simulink model "group2_assignment2_pacemaker_demofile"  (R2023b)
settings: Solver=FixedStepAuto  StartTime=0.0  StopTime=10  FixedStep=1e-3  RelTol=1e-3  EnableMultiTasking=on
model workspace (MAT data in the model file):
  IC = 60
  j = 80
undefined symbols (not defined in the file): D0, D1, D10, D11, D12, D13, D2, D3, D4, D5, D6, D7, D8, D9, PTA0, PTA1, PTA2, PTB23, PTB9, PTC16, PTC17, PTC2, PTC3, PTC4, PTD0, PTD1, PTD2, PTD3
libraries: frdmk64flib x15, dspstat3 x3
settings Model: SimulationMode=external  ExtModeTrigDuration=5  Creator=stivb  LastModifiedBy=bardiased
settings OptimizationCC: EnhancedBackFolding=on  PassReuseOutputArgsAs=Individual arguments  ZeroExternalMemoryAtStartup=off  ZeroInternalMemoryAtStartup=off  MaxStackSize=64  OptimizeBlockOrder=speed  DifferentSizesBufferReuse=on  OptimizationCustomize=off  EfficientTunableParamExpr=on
settings DebuggingCC: ParameterTunabilityLossMsg=error
settings HardwareCC: ProdBitPerPointer=32  ProdBitPerSizeT=32  ProdBitPerPtrDiffT=32  ProdLargestAtomicInteger=Long  ProdLargestAtomicFloat=Double  ProdWordSize=32  ProdHWDeviceType=ARM Compatible->ARM Cortex
settings RTWCC: Description=Embedded Coder  SystemTargetFile=ert.tlc  HardwareBoard=NXP FRDM-K64F  TLCOptions="-aInlineSetEventsForThisBaseRateFcn=TLC_FALSE -aSuppressMultiTaskScheduler=TLC_FALSE  -aRateBasedStepFcn=0"  TemplateMakefile=ert_default_tmf  Toolchain=GNU Tools for ARM Embedded Processors
settings CodeAppCC: ForceParamTrailComments=on  IgnoreCustomStorageClasses=off  OperatorAnnotations=on  SimulinkDataObjDesc=on  SFDataObjDesc=on  InsertBlockDesc=on
settings ERTTargetCC: SupportContinuousTime=on  SupportVariableSizeSignals=on  ExtModeTransport=4  ExtModeMexFile=sendToCommService

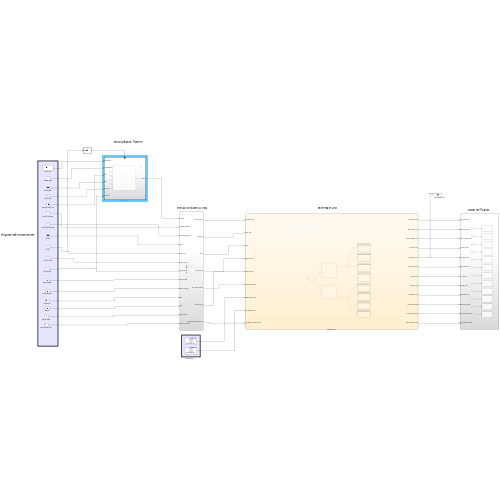
[thumbnail: Simulink's stored preview of the top-level diagram]
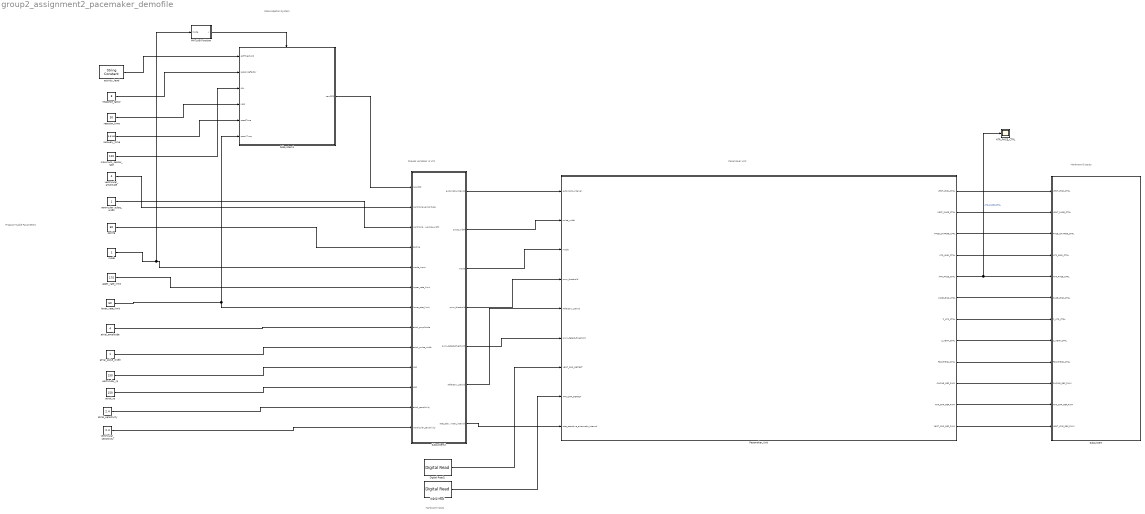
== system group2_assignment2_pacemaker_demofile ==
  note: Rate Adaption System
  note: Hardware inputs
  note: Pseudo variables (4 VM)
  note: Programmable Parameters
  note: Pacemaker Unit
  note: Hardware Outputs
  ATR_PACE_CTRL : Scope
  Digital Read : frdmk64flib/Digital Read  Whichpin=PTC16 (D0)  SampleTime=-1
  Digital Read1 : frdmk64flib/Digital Read  Whichpin=PTC17 (D1)  SampleTime=-1
  MATLAB Function : MATLAB Function  TreatAsAtomicUnit=on
  Pacemaker_Unit : Stateflow chart  TreatAsAtomicUnit=on
      settings: PortSchema="{\"entries\":[{\"content\":{\"sides\":[{\"content\":{\"connectorIds\":[\"In1\",\"In2\",\"In3\",\"In4\",\"In5\",\"In6\",\"In8\",\"In7\",\"In9\"]},\"type\":\"ConnectorPlacement.EquallySpacedRectSide\",\"uuid\":\"c8cba9b3-707c-4f69-ad8c-9d5fbaa12caa\"},{\"content\":{\"connectorIds\":[\"Out1\",\"Out2\",\"Out3\",\"Out4\",\"Out5\",\"Out6\",\"Out7\",\"Out8\",\"Out9\",\"Out10\",\"Out11\",\"Out12\"],\"side\":\"RIGHT\"},\"type\":\"ConnectorPlacement.EquallySpacedRectSide\",\"uuid\":\"918aa1e0-aae1-41d7-a74d-0a72155b1f75\"},{\"content\":{\"side\":\"TOP\"},\"type\":\"ConnectorPlacement.EquallySpacedRectSide\",\"uuid\":\"877803b3-29d8-4e86-807a-7bf9f59cc519\"}]},\"type\":\"ConnectorPlacement.EquallySpacedConnector\",\"uuid\":\"1e148aae-cf3c-4ae1-bc6b-9e679c8c5f2a\"}],\"packageUris\":[\"http://schema.mathworks.com/mf0/Connector/R2020b\"],\"version\":\"1.0\"}"
  Subsystem : Subsystem
  Subsystem1 : Subsystem
  Subsystem2 : Subsystem
  activity_level : StringConstant  String="\"V-Low\""
  atrial_amplitude : Constant  Value=4
  atrial_pulse_width : Constant
  atrial_rp : Constant  Value=150
  atrial_sensitivity : Constant  Value=2.4
  lower_rate_limit : Constant  Value=60
  maximum_sensor_rate : Constant  Value=120
  mode : Constant
  pacing : Constant  Value=60
  reaction_time : Constant  Value=30
  recovery_time : Constant  Value=0.5*60
  response_factor : Constant  Value=8
  upper_rate_limit : Constant  Value=175
  ventricular_amplitude : Constant  Value=4
  ventricular_pulse_width : Constant
  ventricular_rp : Constant  Value=150
  ventricular_sensitivity : Constant  Value=2.4
  wires:
  mode/1 -> MATLAB Function/1(mode), Subsystem2/5(mode_input)
  ventricular_amplitude/1 -> Subsystem2/2(ventricular_amplitude)
  atrial_amplitude/1 -> Subsystem2/8(atrial_amplitude)
  atrial_pulse_width/1 -> Subsystem2/9(atrial_pulse_width)
  lower_rate_limit/1 -> Subsystem1/6(recovTime), Subsystem2/7(lower_rate_limit)
  upper_rate_limit/1 -> Subsystem2/6(upper_rate_limit)
  ventricular_pulse_width/1 -> Subsystem2/3(ventricular_pulse_width)
  pacing/1 -> Subsystem2/4(pacing)
  Subsystem2/1(automatic_interval) -> Pacemaker_Unit/1(automatic_interval)
  Subsystem2/2(pulse_width) -> Pacemaker_Unit/2(pulse_width)
  Subsystem2/3(mode) -> Pacemaker_Unit/3(mode)
  Subsystem2/4(pwm_threshold) -> Pacemaker_Unit/4(pwm_threshold)
  Subsystem2/6(refractory_period) -> Pacemaker_Unit/5(refractory_period)
  Pacemaker_Unit/1(VENT_GND_CTRL) -> Subsystem/1(VENT_GND_CTRL)
  Pacemaker_Unit/2(VENT_PACE_CTRL) -> Subsystem/2(VENT_PACE_CTRL)
  Pacemaker_Unit/3(PACE_CHARGE_CTRL) -> Subsystem/3(PACE_CHARGE_CTRL)
  Pacemaker_Unit/4(ATR_GND_CTRL) -> Subsystem/4(ATR_GND_CTRL)
  Pacemaker_Unit/5(ATR_PACE_CTRL) -> ATR_PACE_CTRL/1, Subsystem/5(ATR_PACE_CTRL)  "ATR_PACE_CTRL"
  Pacemaker_Unit/6(PACE_GND_CTRL) -> Subsystem/6(PACE_GND_CTRL)
  Pacemaker_Unit/7(Z_ATR_CTRL) -> Subsystem/7(Z_ATR_CTRL)
  Pacemaker_Unit/8(Z_VENT_CTRL) -> Subsystem/8(Z_VENT_CTRL)
  Pacemaker_Unit/9(FRONTEND_CTRL) -> Subsystem/9(FRONTEND_CTRL)
  Pacemaker_Unit/10(PACING_REF_PWM) -> Subsystem/10(PACING_REF_PWM)
  ventricular_rp/1 -> Subsystem2/10(VRP)
  atrial_rp/1 -> Subsystem2/11(ARP)
  Pacemaker_Unit/11(ATR_CMP_REF_PWM) -> Subsystem/11(ATR_CMP_REF_PWM)
  Digital Read/1 -> Pacemaker_Unit/7(ATR_CMP_DETECT)
  Digital Read1/1 -> Pacemaker_Unit/8(VENT_CMP_DETECT)
  atrial_sensitivity/1 -> Subsystem2/12(atrial_sensitivity)
  ventricular_sensitivity/1 -> Subsystem2/13(ventricular_sensitivity)
  Subsystem2/5(pwm_detect_threshold) -> Pacemaker_Unit/6(pwm_detect_threshold)
  Pacemaker_Unit/12(VENT_CMP_REF_PWM) -> Subsystem/12(VENT_CMP_REF_PWM)
  Subsystem2/7(rate_adaptive_automatic_interval) -> Pacemaker_Unit/9(rate_adaptive_automatic_interval)
  activity_level/1 -> Subsystem1/1(actThreshold)
  response_factor/1 -> Subsystem1/2(responseFactor)
  maximum_sensor_rate/1 -> Subsystem1/3(LRL)
  reaction_time/1 -> Subsystem1/4(MSR)
  recovery_time/1 -> Subsystem1/5(reactTime)
  Subsystem1/1(newCPR) -> Subsystem2/1(newCPR)
  MATLAB Function/1(y) -> Subsystem1/Enable

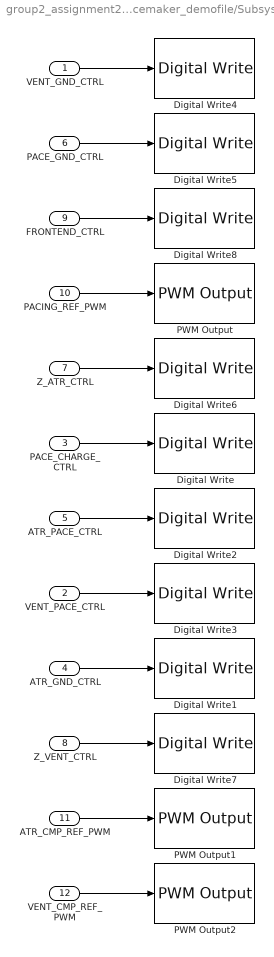
== system group2_assignment2_pacemaker_demofile/Subsystem ==
  VENT_GND_CTRL : Inport
  VENT_PACE_CTRL : Inport  Port=2
  PACE_CHARGE_CTRL : Inport  Port=3
  ATR_GND_CTRL : Inport  Port=4
  ATR_PACE_CTRL : Inport  Port=5
  PACE_GND_CTRL : Inport  Port=6
  Z_ATR_CTRL : Inport  Port=7
  Z_VENT_CTRL : Inport  Port=8
  FRONTEND_CTRL : Inport  Port=9
  PACING_REF_PWM : Inport  Port=10
  ATR_CMP_REF_PWM : Inport  Port=11
  VENT_CMP_REF_PWM : Inport  Port=12
  Digital Write : frdmk64flib/Digital Write  Whichpin=PTB9 (D2)
  Digital Write1 : frdmk64flib/Digital Write  Whichpin=PTD2 (D11)
  Digital Write2 : frdmk64flib/Digital Write  Whichpin=PTA0 (D8)
  Digital Write3 : frdmk64flib/Digital Write  Whichpin=PTC4 (D9)
  Digital Write4 : frdmk64flib/Digital Write  Whichpin=PTD3 (D12)
  Digital Write5 : frdmk64flib/Digital Write  Whichpin=PTD0 (D10)
  Digital Write6 : frdmk64flib/Digital Write  Whichpin=PTB23 (D4)
  Digital Write7 : frdmk64flib/Digital Write  Whichpin=PTC3 (D7)
  Digital Write8 : frdmk64flib/Digital Write  Whichpin=PTD1 (D13)
  PWM Output : frdmk64flib/PWM Output  Whichpin=PTA2 (D5)  InitialFrequency=2000  InitialDutyCycle=0
  PWM Output1 : frdmk64flib/PWM Output  Whichpin=PTC2 (D6)  InitialFrequency=2000  InitialDutyCycle=0
  PWM Output2 : frdmk64flib/PWM Output  Whichpin=PTA1 (D3)  InitialFrequency=2000  InitialDutyCycle=0
  wires:
  Z_ATR_CTRL/1 -> Digital Write6/1
  VENT_PACE_CTRL/1 -> Digital Write3/1
  FRONTEND_CTRL/1 -> Digital Write8/1
  PACING_REF_PWM/1 -> PWM Output/1
  ATR_PACE_CTRL/1 -> Digital Write2/1
  Z_VENT_CTRL/1 -> Digital Write7/1
  VENT_GND_CTRL/1 -> Digital Write4/1
  PACE_CHARGE_CTRL/1 -> Digital Write/1
  ATR_GND_CTRL/1 -> Digital Write1/1
  PACE_GND_CTRL/1 -> Digital Write5/1
  ATR_CMP_REF_PWM/1 -> PWM Output1/1
  VENT_CMP_REF_PWM/1 -> PWM Output2/1

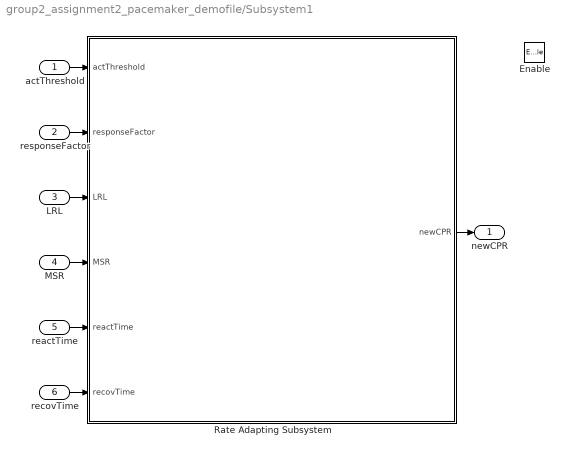
== system group2_assignment2_pacemaker_demofile/Subsystem1 ==
  actThreshold : Inport
  responseFactor : Inport  Port=2
  LRL : Inport  Port=3
  MSR : Inport  Port=4
  reactTime : Inport  Port=5
  recovTime : Inport  Port=6
  Enable : EnablePort
  Rate Adapting Subsystem : Subsystem
  newCPR : Outport
  wires:
  MSR/1 -> Rate Adapting Subsystem/4(MSR)
  reactTime/1 -> Rate Adapting Subsystem/5(reactTime)
  LRL/1 -> Rate Adapting Subsystem/3(LRL)
  Rate Adapting Subsystem/1(newCPR) -> newCPR/1
  responseFactor/1 -> Rate Adapting Subsystem/2(responseFactor)
  recovTime/1 -> Rate Adapting Subsystem/6(recovTime)
  actThreshold/1 -> Rate Adapting Subsystem/1(actThreshold)

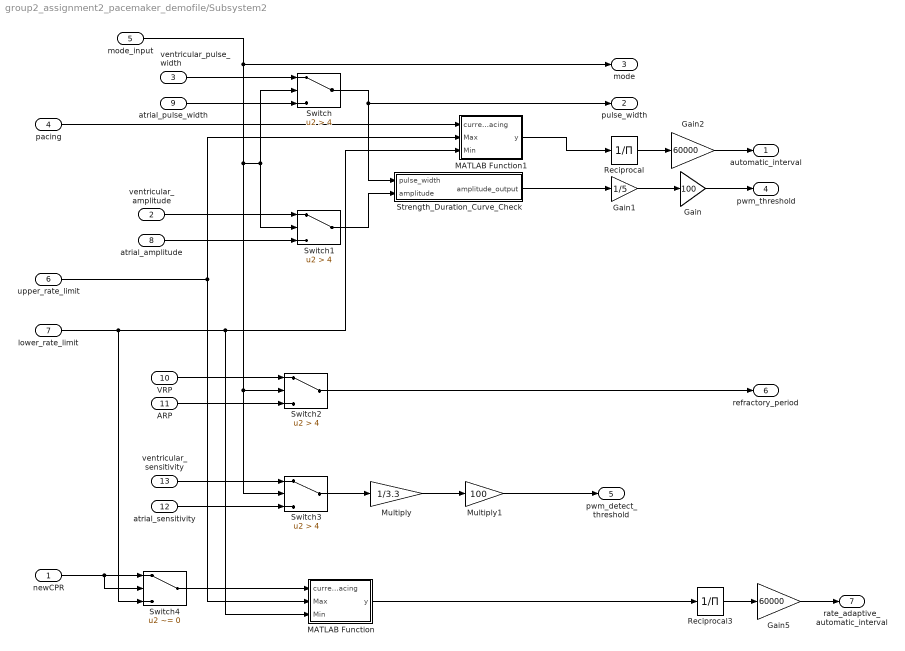
== system group2_assignment2_pacemaker_demofile/Subsystem2 ==
  newCPR : Inport
  ventricular_amplitude : Inport  Port=2
  ventricular_pulse_width : Inport  Port=3
  pacing : Inport  Port=4
  mode_input : Inport  Port=5
  upper_rate_limit : Inport  Port=6
  lower_rate_limit : Inport  Port=7
  atrial_amplitude : Inport  Port=8
  atrial_pulse_width : Inport  Port=9
  VRP : Inport  Port=10
  ARP : Inport  Port=11
  atrial_sensitivity : Inport  Port=12
  ventricular_sensitivity : Inport  Port=13
  Gain : Gain  Gain=100
  Gain1 : Gain  Gain=1/5
  Gain2 : Gain  Gain=60000
  Gain5 : Gain  Gain=60000
  MATLAB Function : MATLAB Function  TreatAsAtomicUnit=on
  MATLAB Function1 : MATLAB Function  TreatAsAtomicUnit=on
  Multiply : Gain  Gain=1/3.3
  Multiply1 : Gain  Gain=100
  Reciprocal : Product  Inputs=/
  Reciprocal3 : Product  Inputs=/
  Strength_Duration_Curve_Check : Stateflow chart  TreatAsAtomicUnit=on
  Switch{,1..3} (4 alike) : Switch  Criteria=u2 > Threshold  Threshold=4  SaturateOnIntegerOverflow=off  InputSameDT=off
  Switch4 : Switch  Criteria=u2 ~= 0  Threshold=4  SaturateOnIntegerOverflow=off  InputSameDT=off
  automatic_interval : Outport
  pulse_width : Outport  Port=2
  mode : Outport  Port=3
  pwm_threshold : Outport  Port=4
  pwm_detect_threshold : Outport  Port=5
  refractory_period : Outport  Port=6
  rate_adaptive_automatic_interval : Outport  Port=7
  wires:
  Gain1/1 -> Gain/1
  upper_rate_limit/1 -> MATLAB Function1/2(Max), MATLAB Function/2(Max)
  Reciprocal/1 -> Gain2/1
  Gain2/1 -> automatic_interval/1
  Gain/1 -> pwm_threshold/1
  Strength_Duration_Curve_Check/1(amplitude_output) -> Gain1/1
  lower_rate_limit/1 -> Switch4/3, MATLAB Function/3(Min), MATLAB Function1/3(Min)
  Switch1/1 -> Strength_Duration_Curve_Check/2(amplitude)
  Switch/1 -> Strength_Duration_Curve_Check/1(pulse_width), pulse_width/1
  Switch2/1 -> refractory_period/1
  VRP/1 -> Switch2/1
  ARP/1 -> Switch2/3
  ventricular_amplitude/1 -> Switch1/1
  ventricular_pulse_width/1 -> Switch/1
  atrial_pulse_width/1 -> Switch/3
  atrial_amplitude/1 -> Switch1/3
  mode_input/1 -> Switch3/2, Switch2/2, Switch1/2, Switch/2, mode/1
  atrial_sensitivity/1 -> Switch3/3
  ventricular_sensitivity/1 -> Switch3/1
  Switch3/1 -> Multiply/1
  Multiply/1 -> Multiply1/1
  Multiply1/1 -> pwm_detect_threshold/1
  Gain5/1 -> rate_adaptive_automatic_interval/1
  Reciprocal3/1 -> Gain5/1
  newCPR/1 -> Switch4/2, Switch4/1
  Switch4/1 -> MATLAB Function/1(currentPacing)
  MATLAB Function/1(y) -> Reciprocal3/1
  pacing/1 -> MATLAB Function1/1(currentPacing)
  MATLAB Function1/1(y) -> Reciprocal/1

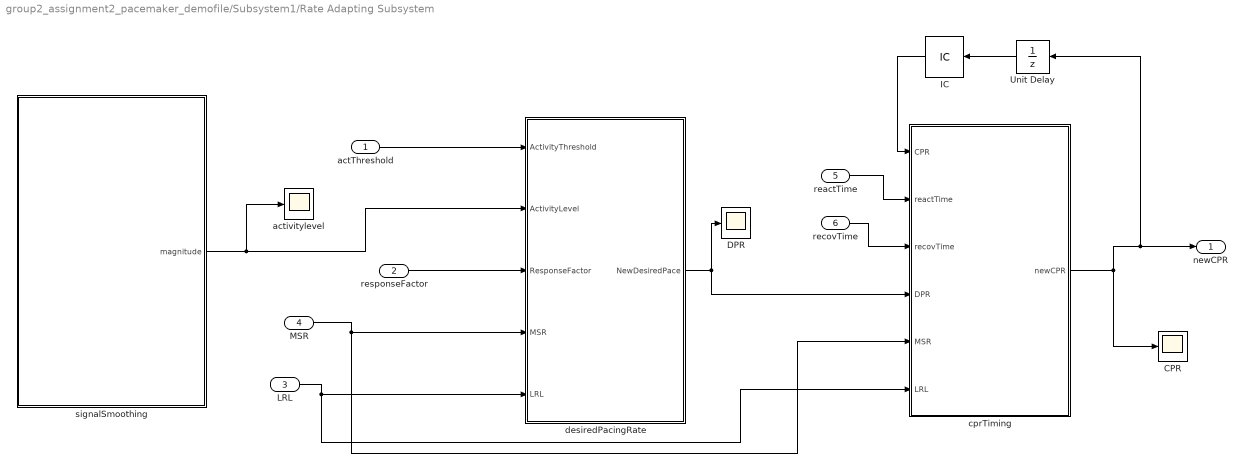
== system group2_assignment2_pacemaker_demofile/Subsystem1/Rate Adapting Subsystem ==
  actThreshold : Inport
  responseFactor : Inport  Port=2
  LRL : Inport  Port=3
  MSR : Inport  Port=4
  reactTime : Inport  Port=5
  recovTime : Inport  Port=6
  CPR : Scope
  DPR : Scope
  IC : InitialCondition  Value=60
  Unit Delay : UnitDelay  SampleTime=-1  HasFrameUpgradeWarning=on
  activitylevel : Scope
  cprTiming : Stateflow chart  TreatAsAtomicUnit=on
  desiredPacingRate : Stateflow chart  TreatAsAtomicUnit=on
  signalSmoothing : Subsystem
  newCPR : Outport
  wires:
  desiredPacingRate/1(NewDesiredPace) -> DPR/1, cprTiming/4(DPR)
  LRL/1 -> desiredPacingRate/5(LRL), cprTiming/6(LRL)
  responseFactor/1 -> desiredPacingRate/3(ResponseFactor)
  MSR/1 -> desiredPacingRate/4(MSR), cprTiming/5(MSR)
  actThreshold/1 -> desiredPacingRate/1(ActivityThreshold)
  cprTiming/1(newCPR) -> Unit Delay/1, newCPR/1, CPR/1
  reactTime/1 -> cprTiming/2(reactTime)
  recovTime/1 -> cprTiming/3(recovTime)
  Unit Delay/1 -> IC/1
  IC/1 -> cprTiming/1(CPR)
  signalSmoothing/1(magnitude) -> activitylevel/1, desiredPacingRate/2(ActivityLevel)

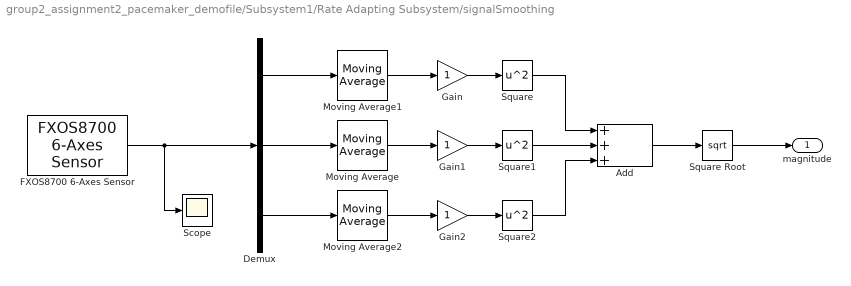
== system group2_assignment2_pacemaker_demofile/Subsystem1/Rate Adapting Subsystem/signalSmoothing ==
  Add : Sum  Inputs=+++
  Demux : Demux  Outputs=3
  FXOS8700 6-Axes Sensor : frdmk64flib/FXOS8700 6-Axes Sensor  Activesensor=Accelerometer only  ODR=800Hz  HybridODR=400Hz  Accelfullrange=-4g to +4g  SampleTime=-1
  Gain : Gain
  Gain1 : Gain
  Gain2 : Gain
  Moving Average : dspstat3/Moving Average  Method=Sliding window  ForgettingFactorPort=off  SpecifyWindowLength=on  WindowLength=4  OverlapLength=3  AllowArbitraryInputLength=off  ForgettingFactor=0.9  SimulateUsing=Code generation
  Moving Average1 : dspstat3/Moving Average  Method=Sliding window  ForgettingFactorPort=off  SpecifyWindowLength=on  WindowLength=4  OverlapLength=3  AllowArbitraryInputLength=off  ForgettingFactor=0.9  SimulateUsing=Code generation
  Moving Average2 : dspstat3/Moving Average  Method=Sliding window  ForgettingFactorPort=off  SpecifyWindowLength=on  WindowLength=4  OverlapLength=3  AllowArbitraryInputLength=off  ForgettingFactor=0.9  SimulateUsing=Code generation
  Scope : Scope
  Square : Math  Operator=square
  Square Root : Sqrt
  Square1 : Math  Operator=square
  Square2 : Math  Operator=square
  magnitude : Outport
  wires:
  Demux/2 -> Moving Average/1
  Moving Average/1 -> Gain1/1
  Demux/1 -> Moving Average1/1
  Moving Average1/1 -> Gain/1
  Demux/3 -> Moving Average2/1
  FXOS8700 6-Axes Sensor/1 -> Scope/1, Demux/1
  Moving Average2/1 -> Gain2/1
  Square Root/1 -> magnitude/1
  Gain/1 -> Square/1
  Gain1/1 -> Square1/1
  Gain2/1 -> Square2/1
  Square/1 -> Add/1
  Square1/1 -> Add/2
  Square2/1 -> Add/3
  Add/1 -> Square Root/1

== stateflow chart group2_assignment2_pacemaker_demofile/Pacemaker_Unit ==
  note: %3CmxGraphModel%3E%3Croot%3E%3CmxCell%20id%3D%220%22%2F%3E%3CmxCell%20id%3D%221%22%20parent%3D%220%22%2F%3E%3CmxCell%20id%3D%222%22%20value%3D%22Assumption%3A%20All%20the%20hazards%20can%20be%20identified%22%20style%3D%22ellipse%3BwhiteSpace%3Dwrap%3Bhtml%3D1%3BfillColor%3D%23CCFFFF%3B%22%20vertex%3D%221%22%20parent%3D%221%22%3E%3CmxGeometry%20x%3D%22370%22%20y%3D%22280%22%20width%3D%22130%22%20height%3D%2280%22%20as%3D%22geometry%22%2F%3E%3C%2FmxCell%3E%3C%2Froot%3E%3C%2FmxGraphModel%3E
  state VOO
    state Charge_C22_Discharge_C21
      entry:
      %Charge C22
      VENT_PACE_CTRL = 0;
      PACE_CHARGE_CTRL = 1;
      %Discharge C21
      VENT_GND_CTRL= 1;
    state ChargeC21_and_DischargeC22
      %Creates the leading edge and sends pulse for X amount of time
      entry:
      PACE_CHARGE_CTRL = 0;
      VENT_GND_CTRL = 0;
      VENT_PACE_CTRL = 1;
      %Recharge pulse is the current in the opposite direction due to C21
    (default) -> VOO.Charge_C22_Discharge_C21
    VOO.Charge_C22_Discharge_C21 -> VOO.ChargeC21_and_DischargeC22 : after(automatic_interval-pulse_width, msec)
    VOO.ChargeC21_and_DischargeC22 -> VOO.Charge_C22_Discharge_C21 : after(pulse_width, msec)
  state VVI
    note: Safe start entry; since hysteresis pacing allows for waiting a period of time longer than the refractory period, we are okay with waiting a refractory period of time before we start pacing. This also ensures that the capacitors are appropriately charged to allow for proper pacing.
    state Refractory_and_charging_ventricle
      entry:
      %Charge C22
      VENT_PACE_CTRL = 0;
      PACE_CHARGE_CTRL = 1;
      %Discharge C21
      VENT_GND_CTRL= 1;
      % Setup sensing pins
      VENT_CMP_REF_PWM = pwm_detect_threshold;
    note: Detected a pace, so go back to refractory state to wait
        | the appropriate refractory time interval
    state Sensing_ventricle
      entry:
      FRONTEND_CTRL = 1;
    state Pacing_ventricle
      entry:
      PACE_CHARGE_CTRL = 0;
      VENT_PACE_CTRL = 1;
      VENT_GND_CTRL = 0;
    (default) -> VVI.Refractory_and_charging_ventricle
    VVI.Refractory_and_charging_ventricle -> VVI.Sensing_ventricle : after(refractory_period, msec)
    VVI.Sensing_ventricle -> VVI.Refractory_and_charging_ventricle [order 1] : [VENT_CMP_DETECT == true]
    VVI.Pacing_ventricle -> VVI.Refractory_and_charging_ventricle : after(pulse_width, msec)
    VVI.Sensing_ventricle -> VVI.Pacing_ventricle [order 2] : after(automatic_interval - refractory_period - pulse_width, msec)
  state Ventricular_Safe_State
    entry: %Safe State
    ATR_PACE_CTRL = 0;
    VENT_PACE_CTRL=0;
    PACING_REF_PWM = pwm_threshold;
    PACE_CHARGE_CTRL=0;
    PACE_GND_CTRL = 1;
    VENT_PACE_CTRL=0;
    Z_ATR_CTRL=0;
    Z_VENT_CTRL=0;
    ATR_PACE_CTRL=0;
    ATR_GND_CTRL=0;
    VENT_GND_CTRL=1;
    FRONTEND_CTRL=0;
  state VOOR
    state Charge_C22_Discharge_C21
      entry:
      %Charge C22
      VENT_PACE_CTRL = 0;
      PACE_CHARGE_CTRL = 1;
      %Discharge C21
      VENT_GND_CTRL= 1;
    state ChargeC21_and_DischargeC22
      %Creates the leading edge and sends pulse for X amount of time
      entry:
      PACE_CHARGE_CTRL = 0;
      VENT_GND_CTRL = 0;
      VENT_PACE_CTRL = 1;
      %Recharge pulse is the current in the opposite direction due to C21
    (default) -> VOOR.Charge_C22_Discharge_C21
    VOOR.Charge_C22_Discharge_C21 -> VOOR.ChargeC21_and_DischargeC22 : after(rate_adaptive_automatic_interval-pulse_width, msec)
    VOOR.ChargeC21_and_DischargeC22 -> VOOR.Charge_C22_Discharge_C21 : after(pulse_width, msec)
  state VVIR
    note: Safe start entry; since hysteresis pacing allows for waiting a period of time longer than the refractory period, we are okay with waiting a refractory period of time before we start pacing. This also ensures that the capacitors are appropriately charged to allow for proper pacing.
    state Refractory_and_charging_ventricle
      entry:
      %Charge C22
      VENT_PACE_CTRL = 0;
      PACE_CHARGE_CTRL = 1;
      %Discharge C21
      VENT_GND_CTRL= 1;
      % Setup sensing pins
      VENT_CMP_REF_PWM = pwm_detect_threshold;
    note: Detected a pace, so go back to refractory state to wait
        | the appropriate refractory time interval
    state Sensing_ventricle
      entry:
      FRONTEND_CTRL = 1;
    state Pacing_ventricle
      entry:
      PACE_CHARGE_CTRL = 0;
      VENT_PACE_CTRL = 1;
      VENT_GND_CTRL = 0;
    (default) -> VVIR.Refractory_and_charging_ventricle
    VVIR.Refractory_and_charging_ventricle -> VVIR.Sensing_ventricle : after(refractory_period, msec)
    VVIR.Sensing_ventricle -> VVIR.Refractory_and_charging_ventricle [order 1] : [VENT_CMP_DETECT == true]
    VVIR.Pacing_ventricle -> VVIR.Refractory_and_charging_ventricle : after(pulse_width, msec)
    VVIR.Sensing_ventricle -> VVIR.Pacing_ventricle [order 2] : after(rate_adaptive_automatic_interval - refractory_period - pulse_width, msec)
  state Mode_Selection
  state AAIR
    note: Safe start entry; since hysteresis pacing allows for waiting a period of time longer than the refractory period, we are okay with waiting a refractory period of time before we start pacing. This also ensures that the capacitors are appropriately charged to allow for proper pacing.
    state Refractory_and_charging_atrial
      entry:
      %Charge C22
      ATR_PACE_CTRL = 0;
      PACE_CHARGE_CTRL = 1;
      %Discharge C21
      ATR_GND_CTRL= 1;
      % Setup sensing pins
      ATR_CMP_REF_PWM = pwm_detect_threshold;
    note: Detected a pace, so go back to refractory state to wait
        | the appropriate refractory time interval
    state Sensing_atrial
      entry:
      FRONTEND_CTRL = 1;
    state Pacing_atrial
      entry:
      PACE_CHARGE_CTRL = 0;
      ATR_PACE_CTRL = 1;
      ATR_GND_CTRL = 0;
    (default) -> AAIR.Refractory_and_charging_atrial
    AAIR.Refractory_and_charging_atrial -> AAIR.Sensing_atrial : after(refractory_period, msec)
    AAIR.Sensing_atrial -> AAIR.Refractory_and_charging_atrial [order 1] : [ATR_CMP_DETECT == true]
    AAIR.Pacing_atrial -> AAIR.Refractory_and_charging_atrial : after(pulse_width, msec)
    AAIR.Sensing_atrial -> AAIR.Pacing_atrial [order 2] : after(rate_adaptive_automatic_interval - refractory_period - pulse_width, msec)
  state Atrial_Safe_State
    entry: %Safe State
    ATR_PACE_CTRL = 0;
    VENT_PACE_CTRL=0;
    PACING_REF_PWM = pwm_threshold;
    PACE_CHARGE_CTRL=0;
    PACE_GND_CTRL = 1;
    VENT_PACE_CTRL=0;
    Z_ATR_CTRL=0;
    Z_VENT_CTRL=0;
    ATR_PACE_CTRL=0;
    ATR_GND_CTRL=1;
    VENT_GND_CTRL=0;
    FRONTEND_CTRL=0;
  state AOOR
    state Charge_C22_Discharge_C21
      entry:
      %Charge C22
      ATR_PACE_CTRL = 0;
      PACE_CHARGE_CTRL = 1;
      %Discharge C21
      ATR_GND_CTRL= 1;
    state ChargeC21_and_DischargeC22
      %Creates the leading edge and sends pulse for X amount of time
      entry:
      PACE_CHARGE_CTRL = 0;
      ATR_PACE_CTRL = 1;
      ATR_GND_CTRL = 0;
    (default) -> AOOR.Charge_C22_Discharge_C21
    AOOR.Charge_C22_Discharge_C21 -> AOOR.ChargeC21_and_DischargeC22 : after(rate_adaptive_automatic_interval-pulse_width, msec)
    AOOR.ChargeC21_and_DischargeC22 -> AOOR.Charge_C22_Discharge_C21 : after(pulse_width, msec)
  state AAI
    note: Safe start entry; since hysteresis pacing allows for waiting a period of time longer than the refractory period, we are okay with waiting a refractory period of time before we start pacing. This also ensures that the capacitors are appropriately charged to allow for proper pacing.
    state Refractory_and_charging_atrial
      entry:
      %Charge C22
      ATR_PACE_CTRL = 0;
      PACE_CHARGE_CTRL = 1;
      %Discharge C21
      ATR_GND_CTRL= 1;
      % Setup sensing pins
      ATR_CMP_REF_PWM = pwm_detect_threshold;
    note: Detected a pace, so go back to refractory state to wait
        | the appropriate refractory time interval
    state Sensing_atrial
      entry:
      FRONTEND_CTRL = 1;
    state Pacing_atrial
      entry:
      PACE_CHARGE_CTRL = 0;
      ATR_PACE_CTRL = 1;
      ATR_GND_CTRL = 0;
    (default) -> AAI.Refractory_and_charging_atrial
    AAI.Refractory_and_charging_atrial -> AAI.Sensing_atrial : after(refractory_period, msec)
    AAI.Sensing_atrial -> AAI.Refractory_and_charging_atrial [order 1] : [ATR_CMP_DETECT == true]
    AAI.Pacing_atrial -> AAI.Refractory_and_charging_atrial : after(pulse_width, msec)
    AAI.Sensing_atrial -> AAI.Pacing_atrial [order 2] : after(automatic_interval - refractory_period - pulse_width, msec)
  state AOO
    state Charge_C22_Discharge_C21
      entry:
      %Charge C22
      ATR_PACE_CTRL = 0;
      PACE_CHARGE_CTRL = 1;
      %Discharge C21
      ATR_GND_CTRL= 1;
    state ChargeC21_and_DischargeC22
      %Creates the leading edge and sends pulse for X amount of time
      entry:
      PACE_CHARGE_CTRL = 0;
      ATR_PACE_CTRL = 1;
      ATR_GND_CTRL = 0;
    (default) -> AOO.Charge_C22_Discharge_C21
    AOO.Charge_C22_Discharge_C21 -> AOO.ChargeC21_and_DischargeC22 : after(automatic_interval-pulse_width, msec)
    AOO.ChargeC21_and_DischargeC22 -> AOO.Charge_C22_Discharge_C21 : after(pulse_width, msec)
  (junction 25) -> VOO [order 1] : [mode == 5]
  (junction 25) -> VVI [order 2] : [mode == 6]
  Ventricular_Safe_State -> (junction 25)
  (junction 25) -> VOOR [order 3] : [mode == 7]
  (junction 25) -> VVIR [order 4] : [mode == 8]
  Mode_Selection -> Ventricular_Safe_State [order 1] : [mode>4]
  (default) -> Mode_Selection
  Mode_Selection -> Atrial_Safe_State [order 2] : [mode <= 4]
  (junction 60) -> AAIR [order 4] : [mode == 4]
  (junction 60) -> AOOR [order 3] : [mode == 3]
  Atrial_Safe_State -> (junction 60)
  (junction 60) -> AAI [order 2] : [mode == 2]
  (junction 60) -> AOO [order 1] : [mode == 1]
  data: automatic_interval input; pulse_width input; mode input; pwm_threshold input; refractory_period input; VENT_GND_CTRL output; VENT_PACE_CTRL output; PACE_CHARGE_CTRL output; ATR_GND_CTRL output; ATR_PACE_CTRL output; PACE_GND_CTRL output; Z_ATR_CTRL output; Z_VENT_CTRL output; FRONTEND_CTRL output; PACING_REF_PWM output; pwm_detect_threshold input; ATR_CMP_DETECT input; ATR_CMP_REF_PWM output; VENT_CMP_DETECT input; VENT_CMP_REF_PWM output; rate_adaptive_automatic_interval input

== stateflow chart group2_assignment2_pacemaker_demofile/Subsystem2/Strength_Duration_Curve_Check ==
  state amplitude_too_low_short_duration
    entry:
    amplitude_output = 4;
  state appropriate_amplitude1
    entry:
    amplitude_output = amplitude;
  state amplitude_too_high_short_duration
    entry:
    amplitude_output = 5;
  state Initalize
  state amplitude_too_low
    entry:
    amplitude_output = 1.6;
  state appropriate_amplitude
    entry:
    amplitude_output = amplitude;
  state amplitude_too_high
    entry:
    amplitude_output = 5;
  (junction 14) -> amplitude_too_low_short_duration [order 2] : [amplitude<4]
  (junction 30) -> appropriate_amplitude1 [order 1] : [amplitude<=5]
  Initalize -> (junction 14) [order 1] : [pulse_width<0.5]
  (junction 14) -> (junction 30) [order 1] : [amplitude>=4]
  (junction 30) -> amplitude_too_high_short_duration [order 2] : [amplitude>5]
  (default) -> Initalize
  Initalize -> (junction 8) [order 2] : [pulse_width>=0.5]
  (junction 8) -> amplitude_too_low [order 2] : [amplitude<1.6]
  (junction 8) -> (junction 22) [order 1] : [amplitude>=1.6]
  (junction 22) -> appropriate_amplitude [order 1] : [amplitude<=5]
  (junction 22) -> amplitude_too_high [order 2] : [amplitude>5]
  data: pulse_width input; amplitude input; amplitude_output output

== matlab function group2_assignment2_pacemaker_demofile/MATLAB Function ==
  data: mode input; y output
function y = fcn(mode)
if(mode==3||mode==4|| mode==7 || mode==8)
    y=1;
else
    y=0;
end

== matlab function group2_assignment2_pacemaker_demofile/Subsystem2/MATLAB Function ==
  data: currentPacing input; y output; Max input; Min input
function y = fcn(currentPacing, Max, Min)

if(currentPacing>Max)
    y = Max;
elseif (currentPacing<Min)
    y = Min;
else
    y= currentPacing;
end

== matlab function group2_assignment2_pacemaker_demofile/Subsystem2/MATLAB Function1 ==
  data: currentPacing input; y output; Max input; Min input
function y = fcn(currentPacing, Max, Min)

if(currentPacing>Max)
    y = Max;
elseif (currentPacing<Min)
    y = Min;
else
    y= currentPacing;
end

== stateflow chart group2_assignment2_pacemaker_demofile/Subsystem1/Rate Adapting Subsystem/cprTiming ==
  state INCREASE_RATE
    entry:
    % Current Time based on Current Pace using inverse function
    currTime = -log(1 - (LRL - CPR)/(LRL - MSR))*(reactTime/11 - 2/11);
    % Increase current time by 1ms
    currTime = currTime + 0.001;
    % New Current Pace Rate after 1ms increase
    newCPR = (1-exp(-11*currTime/(reactTime-2)))*(MSR-LRL) + LRL;
  state INITALIZATION
    entry:
    tolerance = 0.05; %Tolerance to prevent value bouncing
  state DECREASE_RATE
    entry:
    %Current Time based on Current Pace using inverse function
    currTime = -log((LRL - CPR)/(LRL - MSR))*(recovTime/11 - 3/11);
    % Increase current time by 1ms
    currTime = currTime + 0.001;
    %New Current Pace Rate after 1ms increase
    newCPR = (exp(-11*currTime/(recovTime-3)))*(MSR-LRL) + LRL;
  state STABLE
    entry:
    % The rate will not change
    newCPR = CPR;
  INITALIZATION -> INCREASE_RATE [order 1] : [CPR < DPR - tolerance]
  (default) -> INITALIZATION
  INITALIZATION -> DECREASE_RATE [order 2] : [CPR > DPR + tolerance]
  INITALIZATION -> STABLE [order 3] : [(DPR-tolerance)<CPR<(DPR+tolerance)]
  data: CPR input; reactTime input; recovTime input; DPR input; MSR input; LRL input; newCPR output; tolerance local; currTime local

== stateflow chart group2_assignment2_pacemaker_demofile/Subsystem1/Rate Adapting Subsystem/desiredPacingRate ==
  state MaxRate
    %since the activity level is greater than the limit
    %we set out pace at the maximum allowed value
    entry:
    NewDesiredPace = MSR
  state V_Low
    entry:
    activityThresholdNum = 0.05*ATMax+1;
  state Low
    entry:
    activityThresholdNum = 0.15*ATMax+1;
  state DesiredPace
    %activity level is between the max and min limits so we calculate the desired pacing rate using the response factor
    entry:
    NewDesiredPace = (1-exp((-(1/(sqrt(48)-ActivityLevel)*ResponseFactor*(ActivityLevel-activityThresholdNum)))))*(MSR-LRL)+LRL;
  state Med_Low
    entry:
    activityThresholdNum = 0.30*ATMax+1;
  state Definitions
    entry:
    %defining the range of the acceleration values
    %taking into account the baseline by subtracting by 1g
    ATMax = sqrt(4^2+4^2+4^2)-1;
  state Med
    entry:
    activityThresholdNum = 0.45*ATMax+1;
  state MinRate
    %since the activity level is less than the lowest
    %threshold we set out pace at the lowest value
    entry:
    NewDesiredPace = LRL
  state Med_High
    entry:
    activityThresholdNum = 0.60*ATMax+1;
  state High
    entry:
    activityThresholdNum = 0.75*ATMax+1;
  state V_High
    entry:
    activityThresholdNum = 0.90*ATMax+1;
  Definitions -> V_Low [order 1] : [ActivityThreshold == 'V-Low']
  V_Low -> (junction 39)
  (junction 39) -> MaxRate [order 3] : [ActivityLevel > ATMax]
  Definitions -> Low [order 2] : [ActivityThreshold == 'Low']
  Low -> (junction 39)
  (junction 39) -> DesiredPace [order 1] : [ActivityLevel > activityThresholdNum && ActivityLevel  < ATMax]
  (default) -> Definitions
  Med_Low -> (junction 39)
  Definitions -> Med_Low [order 3] : [ActivityThreshold == 'Med-Low']
  Med -> (junction 39)
  (junction 39) -> MinRate [order 2] : [ActivityLevel < activityThresholdNum]
  Med_High -> (junction 39)
  High -> (junction 39)
  V_High -> (junction 39)
  Definitions -> Med [order 4] : [ActivityThreshold == 'Med']
  Definitions -> Med_High [order 5] : [ActivityThreshold == 'Med-High']
  Definitions -> V_High [order 7] : [ActivityThreshold == 'V-High']
  Definitions -> High [order 6] : [ActivityThreshold == 'High']
  data: ActivityThreshold input; ActivityLevel input; ResponseFactor input; MSR input; NewDesiredPace output; LRL input; ATMax local; activityThresholdNum local
